simulink model "controller_arduino"  (R2021b)
settings: Solver=FixedStepAuto  StartTime=0.0  StopTime=inf  FixedStep=1/100  RelTol=1e-3
libraries: arduinolib x8, simulink x2
settings Model: ExtModeTrigDuration=2  Creator=antonio  LastModifiedBy=antonio
settings OptimizationCC: DefaultUnderspecifiedDataType=single  EnhancedBackFolding=on  PassReuseOutputArgsAs=Individual arguments  ZeroExternalMemoryAtStartup=off  ZeroInternalMemoryAtStartup=off  MaxStackSize=64  OptimizeBlockOrder=speed  DifferentSizesBufferReuse=on  OptimizationCustomize=off  EfficientTunableParamExpr=on
settings DebuggingCC: ParameterTunabilityLossMsg=error
settings HardwareCC: ProdBitPerInt=16  ProdBitPerPointer=16  ProdBitPerSizeT=16  ProdBitPerPtrDiffT=16  ProdLargestAtomicFloat=None  ProdWordSize=8  ProdHWDeviceType=Atmel->AVR  UseEmbeddedCoderFeatures=off
settings SFSimCC: MATLABDynamicMemAlloc=off
settings RTWCC: Description=Embedded Coder  SystemTargetFile=ert.tlc  HardwareBoard=Arduino Uno  TemplateMakefile=ert_default_tmf  Toolchain=Arduino AVR
settings CodeAppCC: ForceParamTrailComments=on  IgnoreCustomStorageClasses=off  OperatorAnnotations=on  SimulinkDataObjDesc=on  SFDataObjDesc=on  InsertBlockDesc=on
settings ERTTargetCC: SupportContinuousTime=on  SupportNonInlinedSFcns=on  SupportVariableSizeSignals=on  ExtModeTransport=3  ExtModeStaticAlloc=on  ExtModeStaticAllocSize=250  ExtModeMexFile=ext_xcp  ExtModeIntrfLevel=Level2 - Open
settings ConfigComp: CovEnable=on  RecordCoverage=on  CovModelRefEnable=on

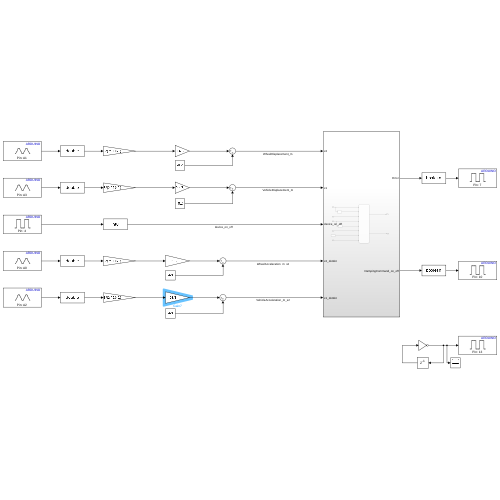
[thumbnail: Simulink's stored preview of the top-level diagram]
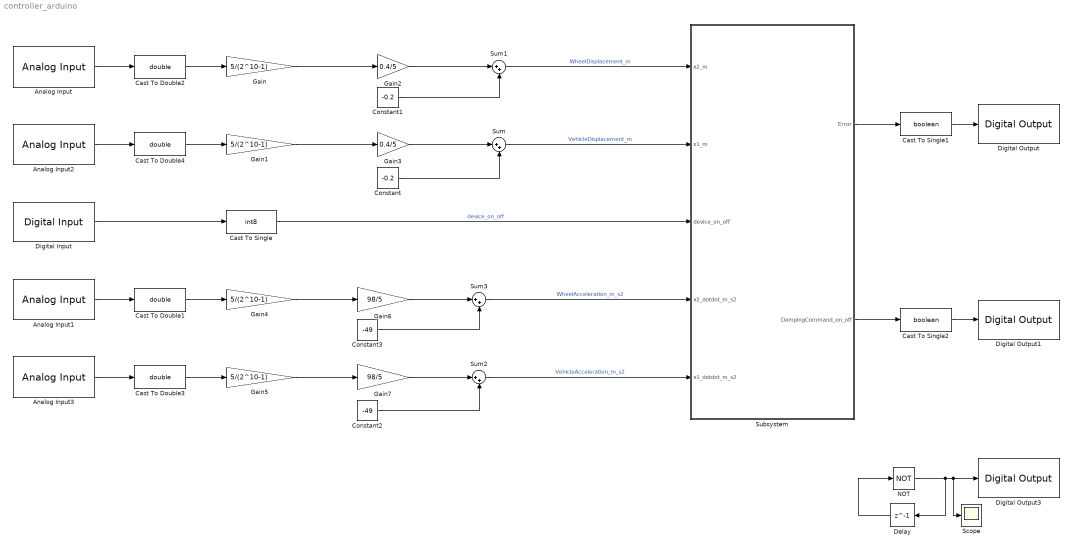
== system controller_arduino ==
  Analog Input : arduinolib/Analog Input  pinNumber=1  ReadResultsOnly=off  ConversionTriggerSource=Software  ExternalTriggerType=uint32( 0 )  OutputDataType=uint16  EnableConversionCompleteNotify=off  EnableOuputStatus=off  SampleTime=1/100  blockPlatform=arduino
  Analog Input1 : arduinolib/Analog Input  pinNumber=0  ReadResultsOnly=off  ConversionTriggerSource=Software  ExternalTriggerType=uint32( 0 )  OutputDataType=uint16  EnableConversionCompleteNotify=off  EnableOuputStatus=off  SampleTime=1/100  blockPlatform=arduino
  Analog Input2 : arduinolib/Analog Input  pinNumber=3  ReadResultsOnly=off  ConversionTriggerSource=Software  ExternalTriggerType=uint32( 0 )  OutputDataType=uint16  EnableConversionCompleteNotify=off  EnableOuputStatus=off  SampleTime=1/100  blockPlatform=arduino
  Analog Input3 : arduinolib/Analog Input  pinNumber=2  ReadResultsOnly=off  ConversionTriggerSource=Software  ExternalTriggerType=uint32( 0 )  OutputDataType=uint16  EnableConversionCompleteNotify=off  EnableOuputStatus=off  SampleTime=1/100  blockPlatform=arduino
  Cast To Double{1..4} (4 alike) : DataTypeConversion  OutDataTypeStr=double
  Cast To Single : DataTypeConversion  OutDataTypeStr=int8
  Cast To Single1 : DataTypeConversion  OutDataTypeStr=boolean
  Cast To Single2 : DataTypeConversion  OutDataTypeStr=boolean
  Constant : Constant  Value=-0.2
  Constant1 : Constant  Value=-0.2
  Constant2 : Constant  Value=-49
  Constant3 : Constant  Value=-49
  Delay : Delay  DelayLength=1  SampleTime=0.5
  Digital Input : arduinolib/Digital Input  pinNumber=4  mode=Default  Direction=input  SampleTime=1/100  blockPlatform=arduino
  Digital Output : arduinolib/Digital Output  pinNumber=7  Direction=output  blockPlatform=arduino
  Digital Output1 : arduinolib/Digital Output  pinNumber=10  Direction=output  blockPlatform=arduino
  Digital Output3 : arduinolib/Digital Output  pinNumber=13  Direction=output  blockPlatform=arduino
  Gain{,1,4..5} (4 alike) : Gain  Gain=5/(2^10-1)
  Gain2 : Gain  Gain=0.4/5
  Gain3 : Gain  Gain=0.4/5
  Gain6 : Gain  Gain=98/5
  Gain7 : Gain  Gain=98/5
  NOT : Logic  Operator=NOT  IconShape=distinctive  AllPortsSameDT=off  OutDataTypeStr=boolean
  Scope : Scope
  Subsystem : Subsystem
  Sum{,1..3} (4 alike) : Sum  Inputs=|++
  wires:
  Subsystem/1(Error) -> Cast To Single1/1
  Subsystem/2(DampingCommand_on_off) -> Cast To Single2/1
  Gain/1 -> Gain2/1
  Digital Input/1 -> Cast To Single/1
  NOT/1 -> Delay/1, Scope/1, Digital Output3/1
  Delay/1 -> NOT/1
  Gain1/1 -> Gain3/1
  Cast To Single/1 -> Subsystem/3(device_on_off)  "device_on_off"
  Cast To Single1/1 -> Digital Output/1
  Cast To Single2/1 -> Digital Output1/1
  Analog Input1/1 -> Cast To Double1/1
  Analog Input3/1 -> Cast To Double3/1
  Analog Input/1 -> Cast To Double2/1
  Cast To Double2/1 -> Gain/1
  Analog Input2/1 -> Cast To Double4/1
  Cast To Double4/1 -> Gain1/1
  Cast To Double1/1 -> Gain4/1
  Cast To Double3/1 -> Gain5/1
  Gain3/1 -> Sum/1
  Sum/1 -> Subsystem/2(x1_m)  "VehicleDisplacement_m"
  Constant/1 -> Sum/2
  Gain2/1 -> Sum1/1
  Sum1/1 -> Subsystem/1(x2_m)  "WheelDisplacement_m"
  Constant1/1 -> Sum1/2
  Sum3/1 -> Subsystem/4(x2_dotdot_m_s2)  "WheelAcceleration_m_s2"
  Gain6/1 -> Sum3/1
  Constant2/1 -> Sum2/2
  Constant3/1 -> Sum3/2
  Sum2/1 -> Subsystem/5(x1_dotdot_m_s2)  "VehicleAcceleration_m_s2"
  Gain7/1 -> Sum2/1
  Gain5/1 -> Gain7/1
  Gain4/1 -> Gain6/1

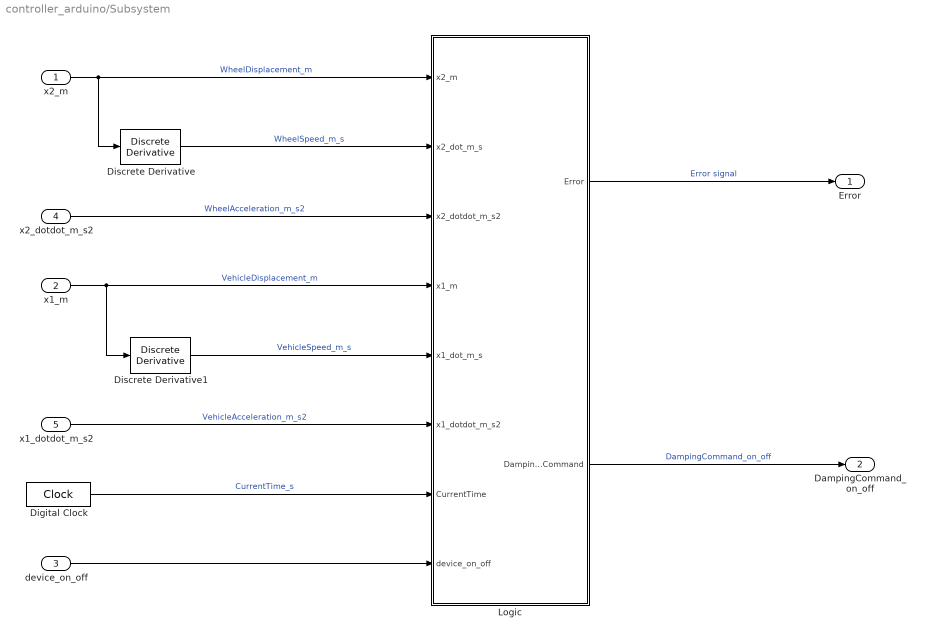
== system controller_arduino/Subsystem ==
  x2_m : Inport  OutDataTypeStr=double
  x1_m : Inport  Port=2
  device_on_off : Inport  Port=3
  x2_dotdot_m_s2 : Inport  Port=4  OutDataTypeStr=double
  x1_dotdot_m_s2 : Inport  Port=5  OutDataTypeStr=double
  Digital Clock : DigitalClock  SampleTime=1/100
  Discrete Derivative : simulink/Discrete/Discrete Derivative  gainval=1.0  ICPrevScaledInput=0.0  OutMin=[]  OutMax=[]  OutDataType=fixdt(1, 16)  OutScaling=2^-10  DoSatur=off
  Discrete Derivative1 : simulink/Discrete/Discrete Derivative  gainval=1.0  ICPrevScaledInput=0.0  OutMin=[]  OutMax=[]  OutDataType=fixdt(1, 16)  OutScaling=2^-10  DoSatur=off
  Logic : Stateflow chart  TreatAsAtomicUnit=on
  Error : Outport  OutDataTypeStr=double
  DampingCommand_on_off : Outport  Port=2  OutDataTypeStr=int8
  wires:
  Logic/2(DampingCommand) -> DampingCommand_on_off/1  "DampingCommand_on_off"
  Discrete Derivative1/1 -> Logic/5(x1_dot_m_s)  "VehicleSpeed_m_s"
  x1_m/1 -> Logic/4(x1_m), Discrete Derivative1/1  "VehicleDisplacement_m"
  x2_m/1 -> Logic/1(x2_m), Discrete Derivative/1  "WheelDisplacement_m"
  Discrete Derivative/1 -> Logic/2(x2_dot_m_s)  "WheelSpeed_m_s"
  Digital Clock/1 -> Logic/7(CurrentTime)  "CurrentTime_s"
  device_on_off/1 -> Logic/8(device_on_off)
  Logic/1(Error) -> Error/1  "Error signal"
  x2_dotdot_m_s2/1 -> Logic/3(x2_dotdot_m_s2)  "WheelAcceleration_m_s2"
  x1_dotdot_m_s2/1 -> Logic/6(x1_dotdot_m_s2)  "VehicleAcceleration_m_s2"

== stateflow chart controller_arduino/Subsystem/Logic ==
  state Device
    state DeviceOff
      entry:
      Error = 0;
      DampingCommand=0;
    state DeviceOn
      during:
      DecisionLogic();
      state Logic [parallel]
        settings: executionOrder=1
        state ControlLogic
          state HighDamping
            entry:
            DampingCommand=1;
          state LowDamping
            entry:
            DampingCommand=0;
          (default) -> HighDamping
          LowDamping -> HighDamping : [DampingStatus == "HiDamping"]
          HighDamping -> LowDamping : [DampingStatus == "LoDamping"]
        ControlLogic -> (junction 135)
        (junction 136) -> ControlLogic : {send(EStop,Warning)}
        (junction 135) -> (junction 136) : [CheckFaultSystem()]
      state Warning [parallel]
        settings: executionOrder=2
        state Running
        state Stop
          entry:
          Error=1;
          DampingCommand=1;
        (default) -> Running
        Running -> Stop : EStop
    (default) -> DeviceOff
    DeviceOn -> DeviceOff : [device_on_off==0]
    DeviceOff -> DeviceOn : [device_on_off==1]
  data: flag function_output; Error output double size=1 [0..1]; x2_m input double size=1; x2_dot_m_s input; x2_dotdot_m_s2 input double size=1; x1_m input double size=1; x1_dot_m_s input; DampingCommand output int8 size=1 [0..1]; x1_dotdot_m_s2 input double size=1; CurrentTime input double; DampingStatus local string; device_on_off input int8
  events: EStop local FUNCTION_CALL_EVENT
  function DecisionLogic:
    | function DecisionLogic
    | 
    | aVarTruthTableCondition_1 = false;
    | aVarTruthTableCondition_2 = false;
    | 
    | 
    | % High damping required
    | 
    | aVarTruthTableCondition_1 = logical((x1_dot_m_s-x2_dot_m_s)*x1_dot_m_s>=0 && Error<1);
    | 
    | % Low damping required
    | 
    | aVarTruthTableCondition_2 = logical((x1_dot_m_s-x2_dot_m_s)*x1_dot_m_s<0 && Error<1);
    | 
    | if (aVarTruthTableCondition_1)
    |     aFcnTruthTableAction_1();
    | elseif (aVarTruthTableCondition_2)
    |     aFcnTruthTableAction_2();
    | else % Default
    |     aFcnTruthTableAction_3();
    | end
    | 
    | function aFcnTruthTableAction_1()
    | 
    | % High damping coefficient
    | 
    | DampingStatus= "HiDamping";
    | 
    | function aFcnTruthTableAction_2()
    | 
    | % Low damping coefficient
    | 
    | DampingStatus = "LoDamping";
    | 
    | function aFcnTruthTableAction_3()
    | 
    | % Nothing
  function flag = CheckFaultSystem:
    | function flag = CheckFaultSystem
    | persistent tol old_x1_dotdot_m_s2 old_x1_m old_x2_m old_x2_dotdot_m_s2 timeChange Error_flag
    | 
    | if isempty(tol)
    |     tol = 1e-8;
    | end
    | 
    | if isempty(Error_flag)
    |     Error_flag = 0;
    | end
    | 
    | if isempty(old_x2_dotdot_m_s2)
    |     old_x2_dotdot_m_s2 = x2_dotdot_m_s2;
    | end
    | 
    | if isempty(old_x2_m)
    |     old_x2_m = x2_m;
    | end
    | 
    | if isempty(old_x1_dotdot_m_s2)
    |     old_x1_dotdot_m_s2 = x1_dotdot_m_s2;
    | end
    | 
    | if isempty(old_x1_m)
    |     old_x1_m = x1_m;
    | end
    | 
    | if isempty(timeChange)
    |     timeChange = CurrentTime;
    | end
    | 
    | if CurrentTime - timeChange >= 0.2 
    |     if abs(old_x1_m-x1_m)<=tol 
    |         Error_flag=1;
    |     elseif abs(old_x2_m-x2_m)<=tol 
    |         Error_flag=1;
    |     elseif abs(old_x1_dotdot_m_s2-x1_dotdot_m_s2)<=tol
    |         Error_flag=1;
    |     elseif abs(old_x2_dotdot_m_s2-x2_dotdot_m_s2)<=tol
    |         Error_flag=1;
    |     end
    |     timeChange = CurrentTime;
    |     old_x1_m = x1_m;
    |     old_x2_m = x2_m;
    |     old_x1_dotdot_m_s2 = x1_dotdot_m_s2;
    |     old_x2_dotdot_m_s2 = x2_dotdot_m_s2;
    |     %disp('%%%%%%%%%%%%%%%%%%%')
    | end
    | 
    | flag=Error_flag;
